simulink model "LCK_old"  (R2018b)
settings: Solver=FixedStepDiscrete  StartTime=0.0  StopTime=inf  FixedStep=0.005  RelTol=1e-3
PostLoadFcn:
  | if any(exist('dsrtsu_mdlpostloadfcn', 'file') ~= 0), dsrtsu_mdlpostloadfcn('Execute', bdroot); end
values from neighbouring files (symbols this model uses):
  C_DEG2RAD = 0.0175    [LCK_Macro.sldd]
  C_KPH2MPS = 0.2778    [LCK_Macro.sldd]
  C_NEARZERO = 0.0001    [LCK_Macro.sldd]
  C_ONE = 1.0    [LCK_Macro.sldd]
  C_RAD2DEG = 57.2958    [LCK_Macro.sldd]
  C_ZERO = 0.0    [LCK_Macro.sldd]
  k_accel_pedal_pos_per_speed_x : value not decoded    [LCK_LogicPara.sldd]
  k_accel_pedal_pos_per_speed_z : value not decoded    [LCK_LogicPara.sldd]
  k_brake_suprress_hold = 1000.0    [LCK_LogicPara.sldd]
  k_driver_appl_torque_filt = 50.0    [LCK_LogicPara.sldd]
  k_driver_suppression_hold_time = 3000.0    [LCK_LogicPara.sldd]
  k_hands_on_wheel_hold_msec = 500.0    [LCK_LogicPara.sldd]
  k_hands_on_wheel_torque_hi = 0.2    [LCK_LogicPara.sldd]
  k_hands_on_wheel_torque_lo = 0.15    [LCK_LogicPara.sldd]
  k_handsoff_delay_cycles = 50.0    [LCK_LogicPara.sldd]
  k_handsoff_torq_Lo_CR = 0.3    [LCK_LogicPara.sldd]
  k_handson_delay_cycles = 5.0    [LCK_LogicPara.sldd]
  k_HighAccel_suppress_hold = 3000.0    [LCK_LogicPara.sldd]
  k_HLR_suprress_hold = 3000.0    [LCK_LogicPara.sldd]
  k_hs_StrAng_CR_threshold_z : value not decoded    [LCK_LogicPara.sldd]
  k_LC_Exit_Switch = 0.0    [LCK_LogicPara.sldd]
  k_LCG_Configured = 1.0    [LCK_LogicPara.sldd]
  k_LCK_A0_Rdy2Act_UseConst = 0.0    [LCK_LogicPara.sldd]
  k_LCK_A0Fac_ActSta : value not decoded    [LCK_CtrlPara.sldd]
  k_LCK_A0Fac_DrvStm : value not decoded    [LCK_CtrlPara.sldd]
  k_LCK_A0Shift_LftCurv : value not decoded    [LCK_CtrlPara.sldd]
  k_LCK_A0Shift_RgtCurv : value not decoded    [LCK_CtrlPara.sldd]
  k_LCK_A0Shift_StraLan = 0.0    [LCK_CtrlPara.sldd]
  k_LCK_A0ShiftFac_Dy_LftCurv : value not decoded    [LCK_CtrlPara.sldd]
  k_LCK_A0ShiftFac_Dy_RgtCurv : value not decoded    [LCK_CtrlPara.sldd]
  k_LCK_A0ShiftFac_Vspd : value not decoded    [LCK_CtrlPara.sldd]
  k_LCK_accel_inhibit_thold = 35.0    [LCK_LogicPara.sldd]
  k_LCK_Active2Ready_Mask = 255.0    [LCK_LogicPara.sldd]
  k_LCK_CvatRateBks : value not decoded    [LCK_CtrlPara.sldd]
  k_LCK_CvatrBks : value not decoded    [LCK_CtrlPara.sldd]
  k_LCK_DFac_Dy : value not decoded    [LCK_CtrlPara.sldd]
  k_LCK_DFac_Dy_Curv : value not decoded    [LCK_CtrlPara.sldd]
  k_LCK_DFac_HaCurCen : value not decoded    [LCK_CtrlPara.sldd]
  k_LCK_DFac_HaCurSid : value not decoded    [LCK_CtrlPara.sldd]
  k_LCK_DFac_HadCurCen : value not decoded    [LCK_CtrlPara.sldd]
  k_LCK_DFac_HadCurSid : value not decoded    [LCK_CtrlPara.sldd]
  k_LCK_DFac_HadStrCen : value not decoded    [LCK_CtrlPara.sldd]
  k_LCK_DFac_HadStrSid : value not decoded    [LCK_CtrlPara.sldd]
  k_LCK_DFac_HaStrCen : value not decoded    [LCK_CtrlPara.sldd]
  k_LCK_DFac_HaStrSid : value not decoded    [LCK_CtrlPara.sldd]
  k_LCK_DFac_Rad : value not decoded    [LCK_CtrlPara.sldd]
  k_LCK_DFac_SA_CurCen : value not decoded    [LCK_CtrlPara.sldd]
  k_LCK_DFac_SA_CurSid : value not decoded    [LCK_CtrlPara.sldd]
  k_LCK_DFac_SA_StrCen : value not decoded    [LCK_CtrlPara.sldd]
  k_LCK_DFac_SA_StrSid : value not decoded    [LCK_CtrlPara.sldd]
  k_LCK_DFac_SS_CurCen : value not decoded    [LCK_CtrlPara.sldd]
  k_LCK_DFac_SS_CurSid : value not decoded    [LCK_CtrlPara.sldd]
  k_LCK_DFac_SS_StrCen : value not decoded    [LCK_CtrlPara.sldd]
  k_LCK_DFac_SS_StrSid : value not decoded    [LCK_CtrlPara.sldd]
  k_LCK_DFac_Vspd : value not decoded    [LCK_CtrlPara.sldd]
  k_LCK_DlyTm_DrvStim = 0.2    [LCK_CtrlPara.sldd]
  k_LCK_DTermMax = 2.0    [LCK_CtrlPara.sldd]
  k_LCK_DyBks_Curv : value not decoded    [LCK_CtrlPara.sldd]
  k_LCK_Enable_POOnly = 1.0    [LCK_LogicPara.sldd]
  k_LCK_Entry_DistBuffer = 0.1    [LCK_LogicPara.sldd]
  k_LCK_Fac_Vspd2RngThr_FalRec = 0.23    [LCK_CtrlPara.sldd]
  k_LCK_Ffw_CvatSwh = 0.0    [LCK_CtrlPara.sldd]
  k_LCK_Ffw_DyBks : value not decoded    [LCK_CtrlPara.sldd]
  k_LCK_Ffw_TimCon_CmdFlt = 0.0    [LCK_CtrlPara.sldd]
  k_LCK_FfwDeltaFac_Rad_Lft : value not decoded    [LCK_CtrlPara.sldd]
  k_LCK_FfwDeltaFac_Rad_Rgt : value not decoded    [LCK_CtrlPara.sldd]
  k_LCK_FfwDeltaFac_Vspd : value not decoded    [LCK_CtrlPara.sldd]
  k_LCK_FfwFac_CvatRate_Lft : value not decoded    [LCK_CtrlPara.sldd]
  k_LCK_FfwFac_CvatRate_Rgt : value not decoded    [LCK_CtrlPara.sldd]
  k_LCK_FfwFac_Dy : value not decoded    [LCK_CtrlPara.sldd]
  k_LCK_FfwFac_Rad_Lft : value not decoded    [LCK_CtrlPara.sldd]
  k_LCK_FfwFac_Rad_Rgt : value not decoded    [LCK_CtrlPara.sldd]
  k_LCK_FfwFac_Vspd : value not decoded    [LCK_CtrlPara.sldd]
  k_LCK_FfwTorq_Cvat : value not decoded    [LCK_CtrlPara.sldd]
  k_LCK_HAFac_ActSta : value not decoded    [LCK_CtrlPara.sldd]
  k_LCK_HAFac_DrvStm : value not decoded    [LCK_CtrlPara.sldd]
  k_LCK_HaloTime = 2000.0    [LCK_LogicPara.sldd]
  k_LCK_HaloTime_Switch = 0.0    [LCK_LogicPara.sldd]
  k_LCK_HARFac_ActSta : value not decoded    [LCK_CtrlPara.sldd]
  k_LCK_HARFac_DrvStm : value not decoded    [LCK_CtrlPara.sldd]
  k_LCK_Hed_DyBks : value not decoded    [LCK_CtrlPara.sldd]
  k_LCK_HedAngDiffX : value not decoded    [LCK_CtrlPara.sldd]
  k_LCK_HedAngRateDiffX : value not decoded    [LCK_CtrlPara.sldd]
  k_LCK_HndsOnWhel_DlyTm_Idl2Rdy = 0.0    [LCK_LogicPara.sldd]
  k_LCK_host_veh_width = 1.86    [LCK_LogicPara.sldd]
  k_LCK_Idle2Ready_Mask = 239.0    [LCK_LogicPara.sldd]
  k_LCK_Junc_SusTime = 1.0    [LCK_LogicPara.sldd]
  k_LCK_KpKdDecSlopeLmt = 10.0    [LCK_CtrlPara.sldd]
  k_LCK_KpKdIncSlopeLmt = 5.0    [LCK_CtrlPara.sldd]
  k_LCK_Lat_Ctrl_DFac_Lft = 1.0    [LCK_CtrlPara.sldd]
  k_LCK_Lat_Ctrl_DFac_Rgt = 1.05    [LCK_CtrlPara.sldd]
  k_LCK_Lat_Ctrl_Kd = 0.8    [LCK_CtrlPara.sldd]
  k_LCK_Lat_Ctrl_Ki = 0.5    [LCK_CtrlPara.sldd]
  k_LCK_Lat_Ctrl_Kp = 0.7    [LCK_CtrlPara.sldd]
  k_LCK_Lat_Ctrl_Kp_NearGain = 0.7    [LCK_CtrlPara.sldd]
  k_LCK_Lat_Ctrl_PFac_Lft = 1.0    [LCK_CtrlPara.sldd]
  k_LCK_Lat_Ctrl_PFac_Rgt = 1.05    [LCK_CtrlPara.sldd]
  k_LCK_Lat_Ctrl_TimCon_CmdFlt = 5.0    [LCK_CtrlPara.sldd]
  k_LCK_Lat_DFac_Rad : value not decoded    [LCK_CtrlPara.sldd]
  k_LCK_Lat_DFac_SS_Cur : value not decoded    [LCK_CtrlPara.sldd]
  k_LCK_Lat_DFac_SS_Str : value not decoded    [LCK_CtrlPara.sldd]
  k_LCK_Lat_DFac_Vspd : value not decoded    [LCK_CtrlPara.sldd]
  k_LCK_Lat_DyBks : value not decoded    [LCK_CtrlPara.sldd]
  k_LCK_Lat_IFac_Rad : value not decoded    [LCK_CtrlPara.sldd]
  k_LCK_Lat_IFac_Vspd : value not decoded    [LCK_CtrlPara.sldd]
  k_LCK_Lat_ILmtFac_Dy_CurvLan : value not decoded    [LCK_CtrlPara.sldd]
  k_LCK_Lat_ILmtFac_Dy_StraLan : value not decoded    [LCK_CtrlPara.sldd]
  k_LCK_Lat_ILmtFac_Rad : value not decoded    [LCK_CtrlPara.sldd]
  k_LCK_Lat_ILmtFac_Rad_NearGain = 1.0    [LCK_CtrlPara.sldd]
  k_LCK_Lat_ILmtFac_Vspd_CurvLan : value not decoded    [LCK_CtrlPara.sldd]
  k_LCK_Lat_ILmtFac_Vspd_StraLan : value not decoded    [LCK_CtrlPara.sldd]
  k_LCK_Lat_ITermLmt_Dy = 1.0    [LCK_CtrlPara.sldd]
  k_LCK_Lat_KpKdDecSlopeLmt = 10.0    [LCK_CtrlPara.sldd]
  k_LCK_Lat_KpKdIncSlopeLmt = 10.0    [LCK_CtrlPara.sldd]
  k_LCK_Lat_PFac_Dy_InnLftCur : value not decoded    [LCK_CtrlPara.sldd]
  k_LCK_Lat_PFac_Dy_InnRgtCur : value not decoded    [LCK_CtrlPara.sldd]
  k_LCK_Lat_PFac_Dy_OutLftCur : value not decoded    [LCK_CtrlPara.sldd]
  k_LCK_Lat_PFac_Dy_OutRgtCur : value not decoded    [LCK_CtrlPara.sldd]
  k_LCK_Lat_PFac_Dy_Str : value not decoded    [LCK_CtrlPara.sldd]
  k_LCK_Lat_PFac_Rad : value not decoded    [LCK_CtrlPara.sldd]
  ... (+158 more)
undefined symbols (not defined in the file or in its folder): k_LCK_CurvBks, K_LCK_SPA0A1A2_LMRngCmp_y
libraries: LateralControl_fcns_lib x58, simulink x22
(part 26 of 45)

== system LCK_old/Lateral_Control_Module/LCK_State_Ctrl/LCK_Mode_Transition/ACTIVE2READY_Magic_Calculation ==
  note: LKATrqOvrlTrqDStat
      | 0: inactive
      | 1: active
      | 2:Temporary inhibit
      | 3:Permanantly failed
  TJA_LatCtrl_Rq : Inport
  LCK_Switch : Inport  Port=2
  veh_speed_kph : Inport  Port=3
  f_driv_override_left : Inport  Port=4
  f_driv_override_right : Inport  Port=5
  f_left_driver_suppression : Inport  Port=6
  f_right_driver_suppression : Inport  Port=7
  LeftLaneChange : Inport  Port=8
  RightLaneChange : Inport  Port=9
  ELK_Mode : Inport  Port=10
  LKATrqOvrlTrqDStat : Inport  Port=11
  YawRate_Over_Threshold : Inport  Port=12
  ACTIVE2READY_Magic : LateralControl_fcns_lib/Bit_To_Integer_16  SystemSampleTime=-1
  Active2ReadyBitwise Operator : simulink/Logic and Bit Operations/Bitwise Operator  Description=_GACA26P3.LCK.000_5_  logicop=AND  UseBitMask=off  NumInputPorts=2  BitMask=k_LCK_Active2Ready_Mask  BitMaskRealWorld=Stored Integer
  Constant1 : Constant  Tag={'output',{'type','Int32'},'date',737237.63746197917}  Description=_GWMAB30P3.LCK.000_35_  Value=0
  Constant39 : Constant  Tag={'output',{'type','Int32'},'date',737237.63746197917}  Description=_GWMAB30P3.LCK.000_35_  Value=0
  Constant42 : Constant  Tag={'output',{'type','Int32'},'date',737237.63746243052}  Description=_GWMAB30P3.LCK.000_38_  Value=0
  Constant43 : Constant  Tag={'output',{'type','Int32'},'date',737237.6374625694}  Description=_GWMAB30P3.LCK.000_39_  Value=0
  Constant44 : Constant  Tag={'output',{'type','Int32'},'date',737237.63746271993}  Description=_GWMAB30P3.LCK.000_40_  Value=0
  Constant45 : Constant  Tag={'output',{'type','Int32'},'date',737237.63746285881}  Description=_GWMAB30P3.LCK.000_41_  Value=0
  Constant46 : Constant  Tag={'output',{'type','Int32'},'date',737237.63746298617}  Description=_GWMAB30P3.LCK.000_42_  Value=0
  Constant47 : Constant  Tag={'output',{'type','Int32'},'date',737237.63746313658}  Description=_GWMAB30P3.LCK.000_43_  Value=0
  Constant55 : Constant  Tag={'output',{'type','Int32'},'date',737292.69766020833}  Description=_GWMAB30P4.LCK.000_120_  Value=2
  Constant70 : Constant  Tag={'output',{'type','Int32'},'date',737462.50906664354}  Description=_GWMH9P4.LCK.000_54_  Value=0
  Data Type Conversion34 : DataTypeConversion  Description=_GWMAB30P4.LCK.000_145_
  Data Type Conversion87 : DataTypeConversion  Description=_GACA26P3.LCK.000_7_  OutDataTypeStr=uint16
  Data Type Conversion91 : DataTypeConversion  OutDataTypeStr=uint16
  Delay_Trig : LateralControl_fcns_lib/Delay_Trig  SystemSampleTime=-1
  ELK_MODE_STAGE1_LEFT1 : Constant  Tag={'output',{'name','$P','class','EXTERN_MACRO','type','ESR_Typedefs/ELK_Mode_T'},'date',737293.52375892363}  Description=_GWMAB30P4.LCK.000_175_  Value=10
  Logical Operator57 : Logic  Tag={'date',737237.63746896992}  Description=_GWMAB30P3.LCK.000_75_  AllPortsSameDT=off  OutDataTypeStr=boolean
  Logical Operator59 : Logic  Tag={'date',737237.63746924768}  Description=_GWMAB30P3.LCK.000_77_  Operator=OR  AllPortsSameDT=off  OutDataTypeStr=boolean
  Logical Operator60 : Logic  Tag={'date',737237.63746940973}  Description=_GWMAB30P3.LCK.000_78_  Operator=OR  AllPortsSameDT=off  OutDataTypeStr=boolean
  Relational Operator13 : RelationalOperator  Tag={'date',737292.697664537}  Description=_GWMAB30P4.LCK.000_181_  OutDataTypeStr=boolean  RndMeth=Nearest
  Relational Operator26 : RelationalOperator  Tag={'date',737237.63747145829}  Description=_GWMAB30P3.LCK.000_89_  Operator===  OutDataTypeStr=boolean  RndMeth=Nearest
  Relational Operator27 : RelationalOperator  Tag={'date',737292.6976654398}  Description=_GWMAB30P4.LCK.000_183_  Operator===  OutDataTypeStr=boolean  RndMeth=Nearest
  Relational Operator51 : RelationalOperator  Tag={'date',737237.63747305551}  Description=_GWMAB30P3.LCK.000_99_  Operator===  OutDataTypeStr=boolean  RndMeth=Nearest
  Relational Operator63 : RelationalOperator  Tag={'date',737237.63747372688}  Description=_GWMAB30P3.LCK.000_102_  Operator===  OutDataTypeStr=boolean  RndMeth=Nearest
  Relational Operator64 : RelationalOperator  Tag={'date',737237.63747385412}  Description=_GWMAB30P3.LCK.000_103_  Operator=>  OutDataTypeStr=boolean  RndMeth=Nearest
  Relational_Operator3 : RelationalOperator  Tag={'date',737237.6374744213}  Description=_GWMAB30P3.LCK.000_106_  Operator=~=  OutDataTypeStr=boolean  RndMeth=Nearest
  Switch16 : Switch  Tag={'output',{'inheritscaling',1},'threshold',{'type','Int32','scalar',1},'date',737243.53952824068}  Description=_GWMAB30P3.LCK.000_117_  Threshold=0.5
  Switch58 : Switch  Tag={'output',{'type','Bool'},'threshold',{'type','Int32'},'date',737463.7890871875}  Description=_GWMH9P4.LCK.000_146_  Criteria=u2 > Threshold  Threshold=0.5
  ZERO4 : Constant  Tag={'output',{'name','$P','class','EXTERN_CONST','type','Bool'},'date',737395.73579394678}  Description=_GWMAB30P3.LCK.000_121_  Value=C_ZERO  SampleTime=-1
  const1 : Constant  Tag={'output',{'type','Int32'},'date',737237.63747829862}  Description=_GWMAB30P3.LCK.000_126_  Value=0
  const2 : Constant  Tag={'output',{'type','Int32'},'date',737237.63747849537}  Description=_GWMAB30P3.LCK.000_127_  Value=0
  const3 : Constant  Tag={'output',{'type','Int32'},'date',737237.63747906254}  Description=_GWMAB30P3.LCK.000_130_  Value=0
  k_LCG_Configured1 : Constant  Tag={'output',{'name','$P','class','EXTERN_CAL','type','Bool'},'date',737462.72274868051}  Description=_GWMH9P4.LCK.000_171_  Value=k_LCG_Configured
  k_LCK_Active2Ready_Mask : Constant  Value=k_LCK_Active2Ready_Mask
  k_LCK_Ovrd_DlyTm_Rdy2Idl1 : Constant  Tag={'output',{'name','$P','class','EXTERN_CAL','type','Float32'},'date',737246.86453446758}  Description=_GWMAB30P3.LCK.000_136_  Value=k_LCK_Ovrd_DlyTm_Rdy2Idl
  k_LCK_VehSpd_TJA_ICA_Bound2 : Constant  Tag={'output',{'name','$P','class','EXTERN_CAL','type','UInt16'},'date',737246.86429184023}  Description=_GWMAB30P3.LCK.000_152_  Value=k_LCK_VehSpd_TJA_ICA_Bound
  ACTIVE2READY_Magic_Out : Outport
  ACTIVE2READY : Outport  Port=2
  wires:
  f_left_driver_suppression/1 -> ACTIVE2READY_Magic/3
  ACTIVE2READY_Magic/1 -> Data Type Conversion87/1
  Relational Operator26/1 -> Logical Operator57/2
  Data Type Conversion34/1 -> Delay_Trig/1
  [TJA_LatCtrl_Rq] -> Relational Operator63/1
  ELK_MODE_STAGE1_LEFT1/1 -> Relational Operator13/2
  Constant39/1 -> ACTIVE2READY_Magic/10
  Data Type Conversion91/1 -> Active2ReadyBitwise Operator/2
  k_LCK_Ovrd_DlyTm_Rdy2Idl1/1 -> Delay_Trig/2
  const2/1 -> Relational Operator51/2
  Relational Operator51/1 -> Logical Operator57/1
  Constant47/1 -> ACTIVE2READY_Magic/15
  Delay_Trig/1 -> ACTIVE2READY_Magic/2
  Relational Operator13/1 -> ACTIVE2READY_Magic/6
  Relational Operator64/1 -> Switch16/2
  const1/1 -> Relational Operator26/2
  Switch58/1 -> ACTIVE2READY_Magic/5
  Constant42/1 -> ACTIVE2READY_Magic/12
  ELK_Mode/1 -> Relational Operator13/1
  f_driv_override_right/1 -> Logical Operator60/2
  Constant70/1 -> Switch58/1
  const3/1 -> Relational Operator63/2
  YawRate_Over_Threshold/1 -> ACTIVE2READY_Magic/8
  Constant45/1 -> ACTIVE2READY_Magic/11
  ZERO4/1 -> Relational_Operator3/2
  Constant46/1 -> ACTIVE2READY_Magic/14
  Switch16/1 -> ACTIVE2READY_Magic/1
  Logical Operator60/1 -> Data Type Conversion34/1
  Logical Operator57/1 -> Switch16/1
  k_LCK_VehSpd_TJA_ICA_Bound2/1 -> Relational Operator64/2
  Constant43/1 -> ACTIVE2READY_Magic/13
  RightLaneChange/1 -> Logical Operator59/2
  Relational Operator27/1 -> ACTIVE2READY_Magic/7
  LeftLaneChange/1 -> Logical Operator59/1
  f_right_driver_suppression/1 -> ACTIVE2READY_Magic/4
  Relational Operator63/1 -> Switch16/3
  Active2ReadyBitwise Operator/1 -> Relational_Operator3/1
  Constant55/1 -> Relational Operator27/2
  Data Type Conversion87/1 -> ACTIVE2READY_Magic_Out/1, Active2ReadyBitwise Operator/1  "TJA_VehInvalid_Magic"
  LKATrqOvrlTrqDStat/1 -> Relational Operator27/1
  k_LCK_Active2Ready_Mask/1 -> Data Type Conversion91/1
  f_driv_override_left/1 -> Logical Operator60/1
  Constant1/1 -> ACTIVE2READY_Magic/9
  Constant44/1 -> ACTIVE2READY_Magic/16
  Relational_Operator3/1 -> ACTIVE2READY/1
  LCK_Switch/1 -> Relational Operator26/1
  Logical Operator59/1 -> Switch58/3
  TJA_LatCtrl_Rq/1 -> [TJA_LatCtrl_Rq], Relational Operator51/1
  k_LCG_Configured1/1 -> Switch58/2
  veh_speed_kph/1 -> Relational Operator64/1
